simulink model "slexAircraftPitchControlExample"  (R2021b)
settings: Solver=ode45  StartTime=0.0  StopTime=60  FixedStep=.01  RelTol=1e-4  AbsTol=1e-6
PreLoadFcn:
  | load slexAircraftPitchControlData.mat
values from neighbouring files (symbols this model uses):
  a = 2.5348    [slexAircraftPitchControlData.mat]
  b = 64.13    [slexAircraftPitchControlData.mat]
  deltat = 0.1    [slexAircraftPitchControlData.mat]
  deltat1 = 0.01    [slexAircraftPitchControlData.mat]
  fden = [1 188.495559215 17765.287922 837169.470368]    [slexAircraftPitchControlData.mat]
  fnum = [0 0 0 837169.470368]    [slexAircraftPitchControlData.mat]
  Ka = 0.677    [slexAircraftPitchControlData.mat]
  Kf = -1.746    [slexAircraftPitchControlData.mat]
  Ki = -3.864    [slexAircraftPitchControlData.mat]
  Kq = 0.8156    [slexAircraftPitchControlData.mat]
  Md = -6.8847    [slexAircraftPitchControlData.mat]
  Mq = -0.6571    [slexAircraftPitchControlData.mat]
  Mw = -0.00592    [slexAircraftPitchControlData.mat]
  Swg = 3    [slexAircraftPitchControlData.mat]
  Ta = 0.05    [slexAircraftPitchControlData.mat]
  Tal = 0.3959    [slexAircraftPitchControlData.mat]
  Ts = 0.1    [slexAircraftPitchControlData.mat]
  Uo = 689.4    [slexAircraftPitchControlData.mat]
  Vto = 690.4    [slexAircraftPitchControlData.mat]
  W1 = 2.971    [slexAircraftPitchControlData.mat]
  W2 = 4.144    [slexAircraftPitchControlData.mat]
  Zd = -63.9979    [slexAircraftPitchControlData.mat]
  Zw = -0.6385    [slexAircraftPitchControlData.mat]
undefined symbols (not defined in the file or in its folder): DiscIntNeverNeededParam
libraries: simulink x3, cstblocks x1
Description:
  | High angle of attack mode for a digital flight control system
settings Model: Creator=The MathWorks, Inc.  LastModifiedBy=The MathWorks, Inc.
settings SolverCC: AutoScaleAbsTol=off  AlgebraicLoopSolver=TrustRegion
settings DataIOCC: ExternalInput=[]  InitialState=[]  SaveFormat=Array  SaveOutput=off  SaveTime=off  ReturnWorkspaceOutputs=off  SignalLoggingName=logsOut
settings OptimizationCC: BlockReduction=off  BooleanDataType=off  ExpressionDepthLimit=2147483647  InitFltsAndDblsToZero=on  LifeSpan=inf
settings DebuggingCC: SaveWithParameterizedLinksMsg=none  CheckExecutionContextPreStartOutputMsg=on  SignalResolutionControl=TryResolveAllWithWarning  MultiTaskDSMMsg=warning  MultiTaskCondExecSysMsg=none  SigSpecEnsureSampleTimeMsg=none  IntegerOverflowMsg=none  FcnCallInpInsideContextMsg=warning  StateNameClashWarn=warning  SFUnexpectedBacktrackingDiag=warning  SFNoUnconditionalDefaultTransitionDiag=warning  SFExecutionAtInitializationDiag=none  SFMachineParentedDataDiag=warning  IntegerSaturationMsg=none  ArithmeticOperatorsInVariantConditions=warning
settings HardwareCC: ProdBitPerPointer=32  ProdBitPerSizeT=32  ProdBitPerPtrDiffT=32  ProdLargestAtomicFloat=None  ProdIntDivRoundTo=Undefined  ProdEndianess=Unspecified  ProdWordSize=32  ProdHWDeviceType=32-bit Generic
settings ModelReferenceCC: PropagateSignalLabelsOutOfModel=off
settings SFSimCC: SimUseLocalCustomCode=off  SimParseCustomCode=off  CustomCodeUndefinedFunction=UseInterfaceOnly
settings RTWCC: GenCodeOnly=on  TemplateMakefile=grt_vc.tmf  RTWUseLocalCustomCode=off
settings CodeAppCC: StateflowObjectComments=on
settings GRTTargetCC: TargetFcnLib=ansi_tfl_tmw.mat  TargetLangStandard=C89/C90 (ANSI)  CombineOutputUpdateFcns=off  GRTInterface=on
settings ConfigComp: CovMetricSettings=dw  CovSaveCumulativeToWorkspaceVar=on  CovSaveSingleToWorkspaceVar=on  CovExternalEMLEnable=off  CovSFcnEnable=off

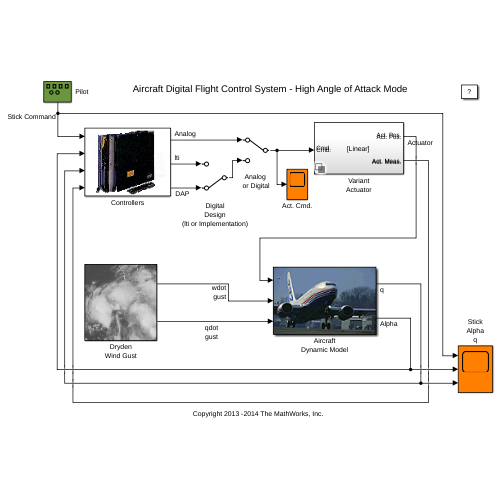
[thumbnail: Simulink's stored preview of the top-level diagram]
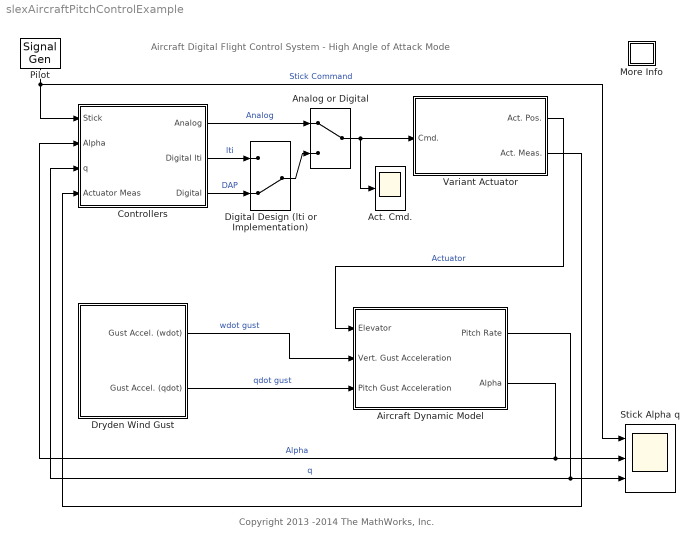
== system slexAircraftPitchControlExample ==
  note: Copyright 2013 -2014 The MathWorks, Inc.
  note: Aircraft Digital Flight Control System - High Angle of Attack Mode
  Act. Cmd. : Scope
  Aircraft Dynamic Model : Subsystem
      mask Display: image('$imagefile'); % Use "Edit Image" on toolstrip to change.
  Analog or Digital : ManualSwitch
  Controllers : Subsystem
      mask Display: image('$imagefile'); % Use "Edit Image" on toolstrip to change.
  Digital Design (lti or Implementation) : ManualSwitch  CurrentSetting=0
  Dryden Wind Gust : Subsystem
      mask Display: image('$imagefile'); % Use "Edit Image" on toolstrip to change.
  More Info : Subsystem
      settings: OpenFcn=showExample('simulink_aerospace/DesigningAHighAngleOfAttackPitchModeControlExample')
      mask Display: disp('?')
  Pilot : SignalGenerator  WaveForm=square  Frequency=.1
  Stick Alpha q : Scope  NumInputPorts=3
  Variant Actuator : Subsystem  Variant=on  VariantControlMode=label  LabelModeActiveChoice=ActuatorType=='Linear'
  wires:
  Controllers/3(Digital) -> Digital Design (lti or Implementation)/2  "DAP"
  Controllers/2(Digital lti) -> Digital Design (lti or Implementation)/1  "lti"
  Digital Design (lti or Implementation)/1 -> Analog or Digital/2
  Variant Actuator/1(Act. Pos.) -> Aircraft Dynamic Model/1(Elevator)  "Actuator"
  Controllers/1(Analog) -> Analog or Digital/1  "Analog"
  Pilot/1 -> Stick Alpha q/1, Controllers/1(Stick)  "Stick Command"
  Aircraft Dynamic Model/2(Alpha) -> Controllers/2(Alpha), Stick Alpha q/2  "Alpha"
  Variant Actuator/2(Act. Meas.) -> Controllers/4(Actuator Meas)
  Dryden Wind Gust/2(Gust Accel. (qdot)) -> Aircraft Dynamic Model/3(Pitch Gust Acceleration)  "qdot gust"
  Dryden Wind Gust/1(Gust Accel. (wdot)) -> Aircraft Dynamic Model/2(Vert. Gust Acceleration)  "wdot gust"
  Aircraft Dynamic Model/1(Pitch Rate) -> Stick Alpha q/3, Controllers/3(q)  "q"
  Analog or Digital/1 -> Variant Actuator/1(Cmd.), Act. Cmd./1

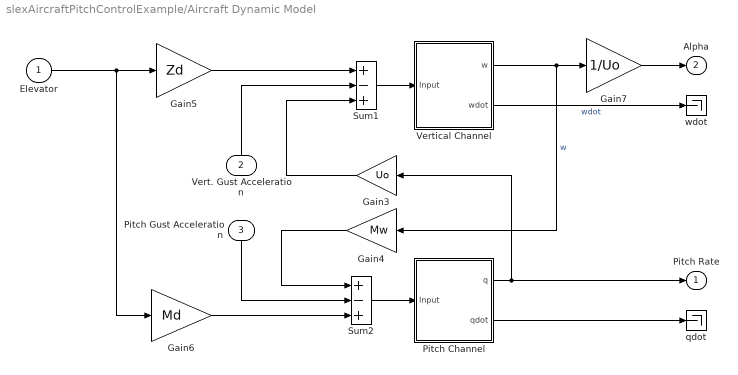
== system slexAircraftPitchControlExample/Aircraft Dynamic Model ==
  Elevator : Inport
  Vert. Gust Acceleration : Inport  Port=2
  Pitch Gust Acceleration : Inport  Port=3
  Gain3 : Gain  Gain=Uo  SaturateOnIntegerOverflow=on  OutDataTypeStr=Inherit: Same as input  ParamDataTypeStr=Inherit: Same as input
  Gain4 : Gain  Gain=Mw  SaturateOnIntegerOverflow=on  OutDataTypeStr=Inherit: Same as input  ParamDataTypeStr=Inherit: Same as input
  Gain5 : Gain  Gain=Zd  SaturateOnIntegerOverflow=on  OutDataTypeStr=Inherit: Same as input  ParamDataTypeStr=Inherit: Same as input
  Gain6 : Gain  Gain=Md  SaturateOnIntegerOverflow=on  OutDataTypeStr=Inherit: Same as input  ParamDataTypeStr=Inherit: Same as input
  Gain7 : Gain  Gain=1/Uo  SaturateOnIntegerOverflow=on  OutDataTypeStr=Inherit: Same as input  ParamDataTypeStr=Inherit: Same as input
  Pitch Channel : Subsystem
  Sum1 : Sum  Inputs=+-+  InputSameDT=on  SaturateOnIntegerOverflow=on  OutDataTypeStr=Inherit: Same as first input
  Sum2 : Sum  Inputs=+-+  InputSameDT=on  SaturateOnIntegerOverflow=on  OutDataTypeStr=Inherit: Same as first input
  Vertical Channel : Subsystem
  qdot : Terminator
  wdot : Terminator
  Pitch Rate : Outport  VectorParamsAs1DForOutWhenUnconnected=off
  Alpha : Outport  Port=2  VectorParamsAs1DForOutWhenUnconnected=off
  wires:
  Pitch Channel/2(qdot) -> qdot/1
  Pitch Channel/1(q) -> Pitch Rate/1, Gain3/1
  Vertical Channel/2(wdot) -> wdot/1  "wdot"
  Vertical Channel/1(w) -> Gain4/1, Gain7/1  "w"
  Sum1/1 -> Vertical Channel/1(Input)
  Gain6/1 -> Sum2/3
  Gain5/1 -> Sum1/1
  Pitch Gust Acceleration/1 -> Sum2/2
  Sum2/1 -> Pitch Channel/1(Input)
  Vert. Gust Acceleration/1 -> Sum1/2
  Elevator/1 -> Gain5/1, Gain6/1
  Gain7/1 -> Alpha/1
  Gain3/1 -> Sum1/3
  Gain4/1 -> Sum2/1

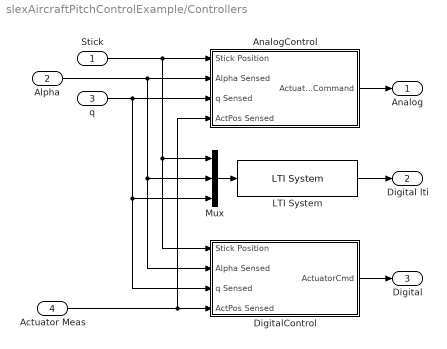
== system slexAircraftPitchControlExample/Controllers ==
  Stick : Inport
  Alpha : Inport  Port=2
  q : Inport  Port=3
  Actuator Meas : Inport  Port=4
  AnalogControl : Subsystem
  DigitalControl : Subsystem
  LTI System : cstblocks/LTI System  sys=discap  IC=[0]
  Mux : Mux  Inputs=3
  Analog : Outport  VectorParamsAs1DForOutWhenUnconnected=off
  Digital lti : Outport  Port=2  VectorParamsAs1DForOutWhenUnconnected=off
  Digital : Outport  Port=3  VectorParamsAs1DForOutWhenUnconnected=off
  wires:
  Stick/1 -> AnalogControl/1(Stick Position), DigitalControl/1(Stick Position), Mux/1
  Actuator Meas/1 -> DigitalControl/4(ActPos Sensed), AnalogControl/4(ActPos Sensed)
  LTI System/1 -> Digital lti/1
  DigitalControl/1(ActuatorCmd) -> Digital/1
  AnalogControl/1(Actuator Command) -> Analog/1
  Mux/1 -> LTI System/1
  Alpha/1 -> AnalogControl/2(Alpha Sensed), DigitalControl/2(Alpha Sensed), Mux/2
  q/1 -> AnalogControl/3(q Sensed), DigitalControl/3(q Sensed), Mux/3

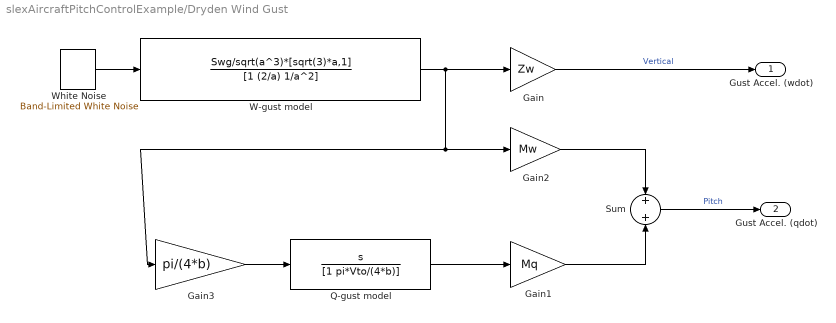
== system slexAircraftPitchControlExample/Dryden Wind Gust ==
  Gain : Gain  Gain=Zw  SaturateOnIntegerOverflow=on  OutDataTypeStr=Inherit: Same as input  ParamDataTypeStr=Inherit: Same as input
  Gain1 : Gain  Gain=Mq  SaturateOnIntegerOverflow=on  OutDataTypeStr=Inherit: Same as input  ParamDataTypeStr=Inherit: Same as input
  Gain2 : Gain  Gain=Mw  SaturateOnIntegerOverflow=on  OutDataTypeStr=Inherit: Same as input  ParamDataTypeStr=Inherit: Same as input
  Gain3 : Gain  Gain=pi/(4*b)  SaturateOnIntegerOverflow=on  OutDataTypeStr=Inherit: Same as input  ParamDataTypeStr=Inherit: Same as input
  Q-gust model : TransferFcn  Numerator=[1 0]  Denominator=[1 pi*Vto/(4*b)]
  Sum : Sum  InputSameDT=on  SaturateOnIntegerOverflow=on  OutDataTypeStr=Inherit: Same as first input
  W-gust model : TransferFcn  Numerator=Swg/sqrt(a^3)*[sqrt(3)*a,1]  Denominator=[1 (2/a) 1/a^2]
  White Noise : simulink/Sources/Band-Limited White Noise  Cov=10  Ts=0.01  seed=23341
  Gust Accel. (wdot) : Outport  VectorParamsAs1DForOutWhenUnconnected=off
  Gust Accel. (qdot) : Outport  Port=2  VectorParamsAs1DForOutWhenUnconnected=off
  wires:
  Gain/1 -> Gust Accel. (wdot)/1  "Vertical"
  White Noise/1 -> W-gust model/1
  Gain3/1 -> Q-gust model/1
  Sum/1 -> Gust Accel. (qdot)/1  "Pitch"
  Gain2/1 -> Sum/1
  Gain1/1 -> Sum/2
  Q-gust model/1 -> Gain1/1
  W-gust model/1 -> Gain/1, Gain2/1, Gain3/1

== system slexAircraftPitchControlExample/More Info ==

== system slexAircraftPitchControlExample/Variant Actuator ==
  Cmd. : Inport
  Linear Actuator Subsystem : Subsystem  VariantControl=ActuatorType=='Linear'
      mask Display: text(0.5,0.5,'[Linear]','horizontalAlignment','center');
  Non-Linear Actuator Subsystem : Subsystem  VariantControl=ActuatorType=='Non-Linear'
      mask Display: text(0.5,0.5,'[Non-Linear]','horizontalAlignment','center')
  Act. Pos. : Outport  VectorParamsAs1DForOutWhenUnconnected=off
  Act. Meas. : Outport  Port=2  VectorParamsAs1DForOutWhenUnconnected=off

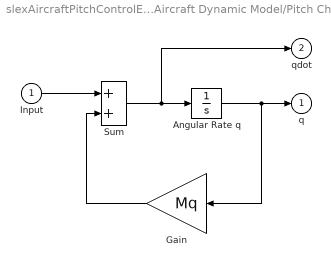
== system slexAircraftPitchControlExample/Aircraft Dynamic Model/Pitch Channel ==
  Input : Inport
  "Angular Rate q " : Integrator
  Gain : Gain  Gain=Mq  SaturateOnIntegerOverflow=on  OutDataTypeStr=Inherit: Same as input  ParamDataTypeStr=Inherit: Same as input
  Sum : Sum  InputSameDT=on  SaturateOnIntegerOverflow=on  OutDataTypeStr=Inherit: Same as first input
  q : Outport  VectorParamsAs1DForOutWhenUnconnected=off
  qdot : Outport  Port=2  VectorParamsAs1DForOutWhenUnconnected=off
  wires:
  Input/1 -> Sum/1
  Gain/1 -> Sum/2
  "Angular Rate q "/1 -> q/1, Gain/1
  Sum/1 -> "Angular Rate q "/1, qdot/1

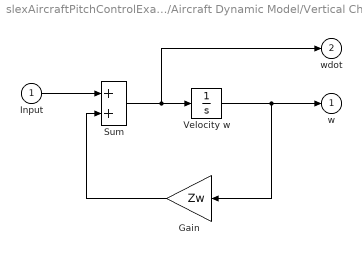
== system slexAircraftPitchControlExample/Aircraft Dynamic Model/Vertical Channel ==
  Input : Inport
  Gain : Gain  Gain=Zw  SaturateOnIntegerOverflow=on  OutDataTypeStr=Inherit: Same as input  ParamDataTypeStr=Inherit: Same as input
  Sum : Sum  InputSameDT=on  SaturateOnIntegerOverflow=on  OutDataTypeStr=Inherit: Same as first input
  Velocity w : Integrator
  w : Outport  VectorParamsAs1DForOutWhenUnconnected=off
  wdot : Outport  Port=2  VectorParamsAs1DForOutWhenUnconnected=off
  wires:
  Sum/1 -> wdot/1, Velocity w/1
  Velocity w/1 -> Gain/1, w/1
  Gain/1 -> Sum/2
  Input/1 -> Sum/1

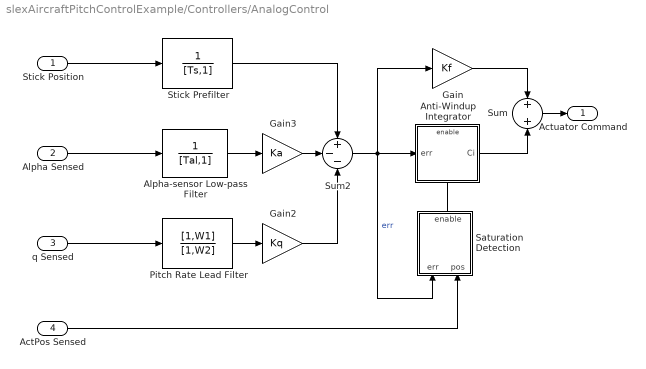
== system slexAircraftPitchControlExample/Controllers/AnalogControl ==
  Stick Position : Inport
  Alpha Sensed : Inport  Port=2
  q Sensed : Inport  Port=3
  ActPos Sensed : Inport  Port=4
  Alpha-sensor Low-pass Filter : TransferFcn  Denominator=[Tal,1]
  Anti-Windup Integrator : Subsystem  TreatAsAtomicUnit=on
      settings: RTWSystemCode=Inline
  Gain : Gain  Gain=Kf  SaturateOnIntegerOverflow=on  OutDataTypeStr=Inherit: Same as input  ParamDataTypeStr=Inherit: Same as input
  Gain2 : Gain  Gain=Kq  SaturateOnIntegerOverflow=on  OutDataTypeStr=Inherit: Same as input  ParamDataTypeStr=Inherit: Same as input
  Gain3 : Gain  Gain=Ka  SaturateOnIntegerOverflow=on  OutDataTypeStr=Inherit: Same as input  ParamDataTypeStr=Inherit: Same as input
  Pitch Rate Lead Filter : TransferFcn  Numerator=[1,W1]  Denominator=[1,W2]
  Saturation Detection : Subsystem
  Stick Prefilter : TransferFcn  Denominator=[Ts,1]
  Sum : Sum  Inputs=2  InputSameDT=on  SaturateOnIntegerOverflow=on  OutDataTypeStr=Inherit: Same as first input
  Sum2 : Sum  Inputs=+--  InputSameDT=on  SaturateOnIntegerOverflow=on  OutDataTypeStr=Inherit: Same as first input
  Actuator Command : Outport  VectorParamsAs1DForOutWhenUnconnected=off
  wires:
  Sum2/1 -> Gain/1, Anti-Windup Integrator/1(err), Saturation Detection/1(err)  "err"
  Anti-Windup Integrator/1(Ci) -> Sum/2
  Sum/1 -> Actuator Command/1
  Stick Position/1 -> Stick Prefilter/1
  Alpha-sensor Low-pass Filter/1 -> Gain3/1
  Gain2/1 -> Sum2/3
  Stick Prefilter/1 -> Sum2/1
  Pitch Rate Lead Filter/1 -> Gain2/1
  Gain3/1 -> Sum2/2
  Gain/1 -> Sum/1
  Alpha Sensed/1 -> Alpha-sensor Low-pass Filter/1
  q Sensed/1 -> Pitch Rate Lead Filter/1
  ActPos Sensed/1 -> Saturation Detection/2(pos)
  Saturation Detection/1(enable) -> Anti-Windup Integrator/Enable

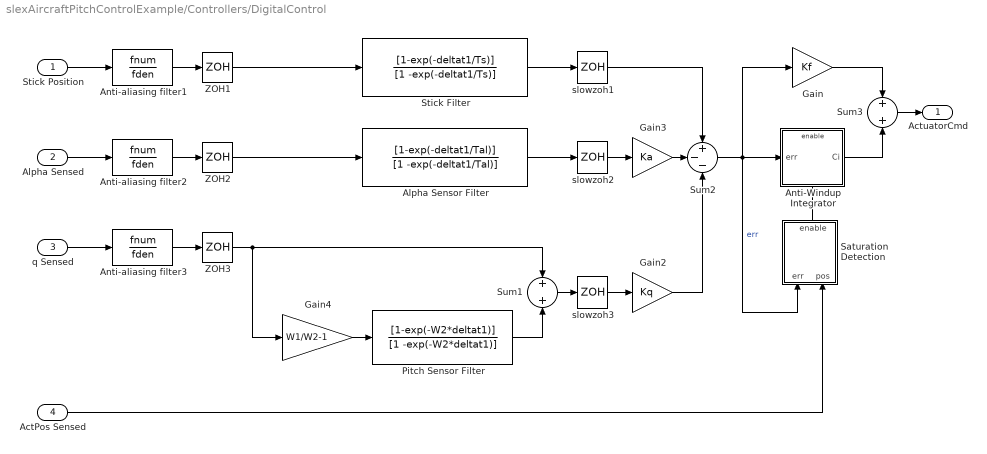
== system slexAircraftPitchControlExample/Controllers/DigitalControl ==
  Stick Position : Inport
  Alpha Sensed : Inport  Port=2
  q Sensed : Inport  Port=3
  ActPos Sensed : Inport  Port=4
  Alpha Sensor Filter : DiscreteTransferFcn  Numerator=[1-exp(-deltat1/Tal)]  Denominator=[1 -exp(-deltat1/Tal)]  SampleTime=deltat1
  Anti-Windup Integrator : Subsystem  TreatAsAtomicUnit=on
      settings: RTWSystemCode=Inline
  Anti-aliasing filter1 : TransferFcn  Numerator=fnum  Denominator=fden
      settings: AttributesFormatString=%<Description>
  Anti-aliasing filter2 : TransferFcn  Numerator=fnum  Denominator=fden
      settings: AttributesFormatString=%<Description>
  Anti-aliasing filter3 : TransferFcn  Numerator=fnum  Denominator=fden
      settings: AttributesFormatString=%<Description>
  Gain : Gain  Gain=Kf  SaturateOnIntegerOverflow=on  OutDataTypeStr=Inherit: Same as input  ParamDataTypeStr=Inherit: Same as input
  Gain2 : Gain  Gain=Kq  SaturateOnIntegerOverflow=on  OutDataTypeStr=Inherit: Same as input  ParamDataTypeStr=Inherit: Same as input
  Gain3 : Gain  Gain=Ka  SaturateOnIntegerOverflow=on  OutDataTypeStr=Inherit: Same as input  ParamDataTypeStr=Inherit: Same as input
  Gain4 : Gain  Gain=W1/W2-1  SaturateOnIntegerOverflow=on  OutDataTypeStr=Inherit: Same as input  ParamDataTypeStr=Inherit: Same as input
  Pitch Sensor Filter : DiscreteTransferFcn  Numerator=[1-exp(-W2*deltat1)]  Denominator=[1 -exp(-W2*deltat1)]  SampleTime=deltat1
  Saturation Detection : Subsystem
  Stick Filter : DiscreteTransferFcn  Numerator=[1-exp(-deltat1/Ts)]  Denominator=[1 -exp(-deltat1/Ts)]  SampleTime=deltat1
  Sum1 : Sum  Inputs=2  InputSameDT=on  SaturateOnIntegerOverflow=on  OutDataTypeStr=Inherit: Same as first input
  Sum2 : Sum  Inputs=+--  InputSameDT=on  SaturateOnIntegerOverflow=on  OutDataTypeStr=Inherit: Same as first input
  Sum3 : Sum  Inputs=2  InputSameDT=on  SaturateOnIntegerOverflow=on  OutDataTypeStr=Inherit: Same as first input
  ZOH1 : ZeroOrderHold  SampleTime=deltat1
  ZOH2 : ZeroOrderHold  SampleTime=deltat1
  ZOH3 : ZeroOrderHold  SampleTime=deltat1
  slowzoh1 : ZeroOrderHold  SampleTime=deltat
  slowzoh2 : ZeroOrderHold  SampleTime=deltat
  slowzoh3 : ZeroOrderHold  SampleTime=deltat
  ActuatorCmd : Outport  VectorParamsAs1DForOutWhenUnconnected=off
  wires:
  Sum3/1 -> ActuatorCmd/1
  Sum2/1 -> Gain/1, Anti-Windup Integrator/1(err), Saturation Detection/1(err)  "err"
  Alpha Sensed/1 -> Anti-aliasing filter2/1
  Stick Filter/1 -> slowzoh1/1
  slowzoh1/1 -> Sum2/1
  Alpha Sensor Filter/1 -> slowzoh2/1
  slowzoh2/1 -> Gain3/1
  Gain3/1 -> Sum2/2
  Gain/1 -> Sum3/1
  Anti-Windup Integrator/1(Ci) -> Sum3/2
  Gain2/1 -> Sum2/3
  q Sensed/1 -> Anti-aliasing filter3/1
  Sum1/1 -> slowzoh3/1
  Pitch Sensor Filter/1 -> Sum1/2
  Gain4/1 -> Pitch Sensor Filter/1
  slowzoh3/1 -> Gain2/1
  Stick Position/1 -> Anti-aliasing filter1/1
  ZOH1/1 -> Stick Filter/1
  Anti-aliasing filter1/1 -> ZOH1/1
  Anti-aliasing filter2/1 -> ZOH2/1
  Anti-aliasing filter3/1 -> ZOH3/1
  ZOH2/1 -> Alpha Sensor Filter/1
  ZOH3/1 -> Sum1/1, Gain4/1
  Saturation Detection/1(enable) -> Anti-Windup Integrator/Enable
  ActPos Sensed/1 -> Saturation Detection/2(pos)

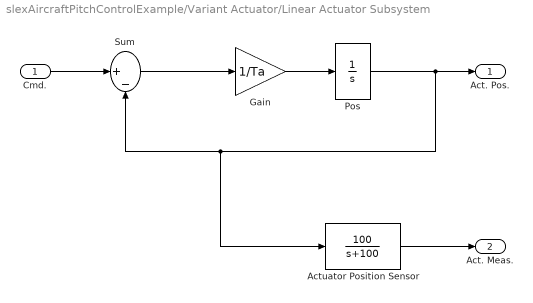
== system slexAircraftPitchControlExample/Variant Actuator/Linear Actuator Subsystem ==
  Cmd. : Inport
  Actuator Position Sensor : TransferFcn  Numerator=[100]  Denominator=[1 100]
  Gain : Gain  Gain=1/Ta  SaturateOnIntegerOverflow=on  OutDataTypeStr=Inherit: Same as input  ParamDataTypeStr=Inherit: Same as input
  Pos : Integrator  UpperSaturationLimit=pi*45/180  LowerSaturationLimit=-pi*45/180
  Sum : Sum  Inputs=|+-  InputSameDT=on  SaturateOnIntegerOverflow=on  OutDataTypeStr=Inherit: Same as first input
  Act. Pos. : Outport  InitialOutput=0  VectorParamsAs1DForOutWhenUnconnected=off
  Act. Meas. : Outport  Port=2  InitialOutput=0  VectorParamsAs1DForOutWhenUnconnected=off
  wires:
  Actuator Position Sensor/1 -> Act. Meas./1
  Cmd./1 -> Sum/1
  Pos/1 -> Act. Pos./1, Actuator Position Sensor/1, Sum/2
  Gain/1 -> Pos/1
  Sum/1 -> Gain/1

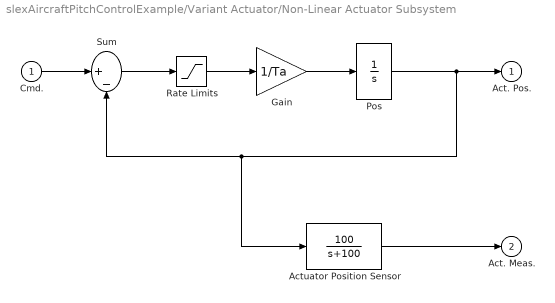
== system slexAircraftPitchControlExample/Variant Actuator/Non-Linear Actuator Subsystem ==
  Cmd. : Inport
  Actuator Position Sensor : TransferFcn  Numerator=[100]  Denominator=[1 100]
  Gain : Gain  Gain=1/Ta  SaturateOnIntegerOverflow=on  OutDataTypeStr=Inherit: Same as input  ParamDataTypeStr=Inherit: Same as input
  Pos : Integrator  LimitOutput=on  UpperSaturationLimit=pi*45/180  LowerSaturationLimit=-pi*45/180
  Rate Limits : Saturate
  Sum : Sum  Inputs=|+-  InputSameDT=on  SaturateOnIntegerOverflow=on  OutDataTypeStr=Inherit: Same as first input
  Act. Pos. : Outport  InitialOutput=0  VectorParamsAs1DForOutWhenUnconnected=off
  Act. Meas. : Outport  Port=2  InitialOutput=0  VectorParamsAs1DForOutWhenUnconnected=off
  wires:
  Actuator Position Sensor/1 -> Act. Meas./1
  Pos/1 -> Act. Pos./1, Actuator Position Sensor/1, Sum/2
  Cmd./1 -> Sum/1
  Sum/1 -> Rate Limits/1
  Gain/1 -> Pos/1
  Rate Limits/1 -> Gain/1

== system slexAircraftPitchControlExample/Controllers/AnalogControl/Anti-Windup Integrator ==
  err : Inport
  Enable : EnablePort
  Gain1 : Gain  Gain=Ki  SaturateOnIntegerOverflow=on  OutDataTypeStr=Inherit: Same as input  ParamDataTypeStr=Inherit: Same as input
  Integrator : Integrator
  Ci : Outport  InitialOutput=0  VectorParamsAs1DForOutWhenUnconnected=off
  wires:
  err/1 -> Integrator/1
  Integrator/1 -> Gain1/1
  Gain1/1 -> Ci/1

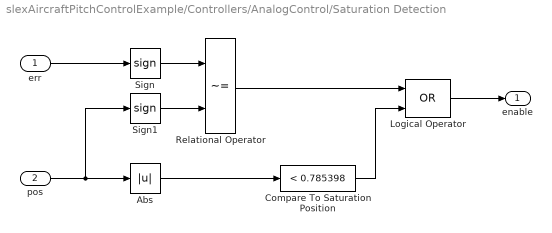
== system slexAircraftPitchControlExample/Controllers/AnalogControl/Saturation Detection ==
  err : Inport
  pos : Inport  Port=2
  Abs : Abs  ZeroCross=off
  Compare To Saturation Position : simulink/Logic and Bit Operations/Compare To Constant  relop=<  const=0.785398  OutDataTypeStr=boolean  ZeroCross=off
  Logical Operator : Logic  Operator=OR  AllPortsSameDT=off  OutDataTypeStr=boolean
  Relational Operator : RelationalOperator  Operator=~=  OutDataTypeStr=boolean  ZeroCross=off  RndMeth=Nearest
  Sign : Signum  ZeroCross=off
  Sign1 : Signum  ZeroCross=off
  enable : Outport  VectorParamsAs1DForOutWhenUnconnected=off
  wires:
  pos/1 -> Sign1/1, Abs/1
  Sign/1 -> Relational Operator/1
  Relational Operator/1 -> Logical Operator/1
  Compare To Saturation Position/1 -> Logical Operator/2
  Sign1/1 -> Relational Operator/2
  Abs/1 -> Compare To Saturation Position/1
  err/1 -> Sign/1
  Logical Operator/1 -> enable/1

== system slexAircraftPitchControlExample/Controllers/DigitalControl/Anti-Windup Integrator ==
  err : Inport
  Enable : EnablePort
  Discrete-Time Integrator : DiscreteIntegrator  IntegratorMethod=Integration: Trapezoidal  SampleTime=deltat  ICPrevOutput=DiscIntNeverNeededParam  ICPrevScaledInput=DiscIntNeverNeededParam
  Gain1 : Gain  Gain=Ki  SaturateOnIntegerOverflow=on  OutDataTypeStr=Inherit: Same as input  ParamDataTypeStr=Inherit: Same as input
  Ci : Outport  InitialOutput=0  VectorParamsAs1DForOutWhenUnconnected=off
  wires:
  err/1 -> Discrete-Time Integrator/1
  Discrete-Time Integrator/1 -> Gain1/1
  Gain1/1 -> Ci/1

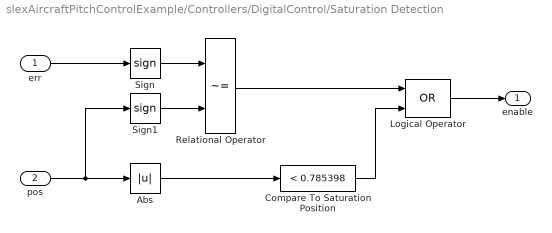
== system slexAircraftPitchControlExample/Controllers/DigitalControl/Saturation Detection ==
  err : Inport
  pos : Inport  Port=2
  Abs : Abs  ZeroCross=off
  Compare To Saturation Position : simulink/Logic and Bit Operations/Compare To Constant  relop=<  const=0.785398  OutDataTypeStr=boolean  ZeroCross=off
  Logical Operator : Logic  Operator=OR  AllPortsSameDT=off  OutDataTypeStr=boolean
  Relational Operator : RelationalOperator  Operator=~=  OutDataTypeStr=boolean  ZeroCross=off  RndMeth=Nearest
  Sign : Signum  ZeroCross=off
  Sign1 : Signum  ZeroCross=off
  enable : Outport  VectorParamsAs1DForOutWhenUnconnected=off
  wires:
  pos/1 -> Sign1/1, Abs/1
  Sign/1 -> Relational Operator/1
  Relational Operator/1 -> Logical Operator/1
  Compare To Saturation Position/1 -> Logical Operator/2
  Sign1/1 -> Relational Operator/2
  Abs/1 -> Compare To Saturation Position/1
  err/1 -> Sign/1
  Logical Operator/1 -> enable/1
